simulink model "DC_Microgrid_Sim"  (R2023b)
settings: Solver=VariableStepDiscrete  StartTime=0.0  StopTime=72  MaxStep=1e-2  RelTol=1e-3
undefined symbols (not defined in the file or in its folder): dEgdT, EgRef, gcbh, Ion, k1, Lithium, Rsh_array5pc, sps_rtmsupport, Tref_K, Tsf, VT_ref
libraries: spsSeriesRLCBranchLib x7, spsVoltageMeasurementLib x5, SignalEditorBlockLib x2, spsCurrentMeasurementLib x2, spsDiodeLib x2, spsFirstOrderFilterLib x2, spsControlledCurrentSourceLib x2, spsPVarrayModel x2, spsBatteryLib x1, spsVariableResistorLib x1, spsBoostConverterLib x1, spsStairGeneratorLib x1
(part 2 of 9)

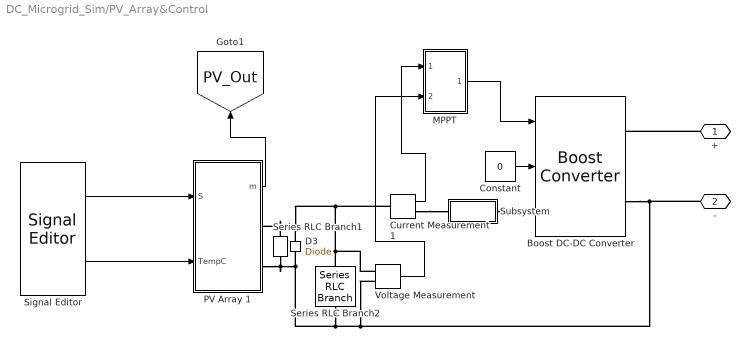
== system DC_Microgrid_Sim/PV_Array&Control ==
  Boost DC-DC Converter : spsBoostConverterLib/Boost Converter  ModelType=Switching function  Ron=1e-3  Rs=1e6  Cs=inf  Vforward=[0,0]  Ron_Diode=1e-3  Rs_Diode=1e6  Cs_Diode=inf  Vf_Diode=0  Rs_CurrentSource=inf  Ron_ACsource=1e-3
  Constant : Constant  Value=0
  Current Measurement1 : spsCurrentMeasurementLib/Current Measurement  PhasorSimulation=off  OutputType=Complex  PSBequivalent=0
  D3 : spsDiodeLib/Diode  Ron=1e-3  Lon=0  Vf=.6  IC=0  UseSnubber=0  Rs=1e6  Cs=inf  Measurements=off
  MPPT : Subsystem
  PV Array 1 : Subsystem  AncestorBlock=spsPVArrayLib/PV Array  DialogController=POWERSYS.PowerSysDialog  LoadFcn=sps_rtmsupport('LoadFcn',gcbh);  StartFcn=sps_rtmsupport('StartFcn',gcbh);  StopFcn=sps_rtmsupport('StopFcn',gcbh);  mask(PV array){Npar=101, Nser=3, PlotType=one module @ 25 deg.C & specified irradiances, S_vec=[ 1000  500  100 ], Temp_C_vec=[ 45 25  ], ModuleName=SunPower SPR-315E-WHT-D, PlotWhenSelected=off, Pm=315.072, Ncell=96, Voc=64.6, Isc=6.14, Vm=54.7, Im=5.76, beta_Voc_pc=-0.2727, alpha_Isc_pc=0.061743, beta_Voc=-0.17616, alpha_Isc=0.003791, IL=6.1461, I0=6.5067e-12, nI=0.95071, Rsh=430.0666, Rs=0.43041, RobustModel=off, RobustCellTemperature=40, BAL=on, Tc=1e-6, Tfilter=5e-5}
      mask prompts: Npar "Parallel strings"; Nser "Series-connected modules per string"; S_vec "Irradiances (W/m2)"; Temp_C_vec "T_cell (deg. C)"; ModuleName "Module:"; PlotWhenSelected "Plot I-V and P-V characteristics when a module is selected"; Pm "Maximum Power (W)"; Ncell "Cells per module (Ncell)"; Voc "Open circuit voltage  Voc (V)"; Isc "Short-circuit current Isc (A)"; Vm "Voltage at maximum power point Vmp (V)"; Im "Current at maximum power point Imp (A)"; beta_Voc_pc "Temperature coefficient of Voc (%/deg.C)"; alpha_Isc_pc "Temperature coefficient of Isc (%/deg.C)"; beta_Voc "Temperature coefficient of Voc (V/deg.C)"; alpha_Isc "Temperature coefficient of Isc (A/deg.C)"; IL "Light-generated current IL (A)"; I0 "Diode saturation current I0 (A)"; nI "Diode ideality factor"; Rsh "Shunt resistance Rsh (ohms)"; Rs "Series resistance Rs (ohms)"; RobustModel "Robust discrete model"; RobustCellTemperature "Cell temperature, in deg.C. (input 2 is disabled)"; BAL "Break algebraic loop in internal model"; Tc "Break loop time constant (s)"; Tfilter "Measurement filter time constant (s)"
      mask help:
      | Implements a PV array built of strings of PV modules connected in parallel. Each string consists of modules connected in series.
      | Allows modeling of a variety of preset PV modules available from NREL System Advisor Model (Jan. 2014) as well as user-defined PV module.
      |
      | Input 1 = Sun irradiance, in W/m2, and input 2 = Cell temperature, in deg.C.
      mask init:
      | Block = gcb;
      | [k,k1,q,Tref_C,Tref_K,EgRef,dEgdT,Rsh_array5pc,VT_ref,Tsf,Tf,VIdiodePV,WantBlockChoice] = PVArrayInit(Block, Nser, Npar, Ncell, Rsh, nI, Tfilter, Voc, I0);
      | powericon('SetInternalModels','set',Block,WantBlockChoice);
      | sps_rtmsupport('parametereditingmodes',Block, [3 6 7 23]);
      settings: CopyFcn=sps_rtmsupport('CopyFcn',gcbh);  DeleteFcn=sps_rtmsupport('DeleteFcn',gcbh);  UndoDeleteFcn=sps_rtmsupport('UndoDeleteFcn',gcbh);  ModelCloseFcn=sps_rtmsupport('ModelCloseFcn',gcbh);  PreSaveFcn=sps_rtmsupport('PreSaveFcn',gcbh);  PostSaveFcn=sps_rtmsupport('PostSaveFcn',gcbh);  NameChangeFcn=sps_rtmsupport('NameChangeFcn',gcbh);  PreCopyFcn=sps_rtmsupport('PreCopyFcn',gcbh);  CloseFcn=sps_rtmsupport('CloseFcn',gcbh);  PreDeleteFcn=sps_rtmsupport('PreDeleteFcn',gcbh);
      settings: OpenFcn=|
      | %assignin('base','PVMaskOpening',1);
      | %open_system(gcb,'mask')
      | %assignin('base','PVMaskOpening',0);
      | sps_rtmsupport('OpenFcn',gcbh, [3 6 7 23]);
      mask Help: helpview(psbhelp);
      mask TypeOptions PlotType: one module @ 25 deg.C & specified irradiances | array @ 25 deg.C & specified irradiances | array @ 1000 W/m2 & specified temperatures
      mask Callback PlotType: PVArrayCback(gcb)
